simulink model "heading_angle_hold_autopilot"  (R2018b)
settings: Solver=VariableStepAuto  StartTime=0.0  StopTime=40  RelTol=1e-3
values from neighbouring files (symbols this model uses):
  g = 32.2    [heading_angle_hold_autopilot.m]
  V = 876    [heading_angle_hold_autopilot.m]
libraries: cstblocks x1
settings Model: Creator=FARYAL  LastModifiedBy=FARYAL

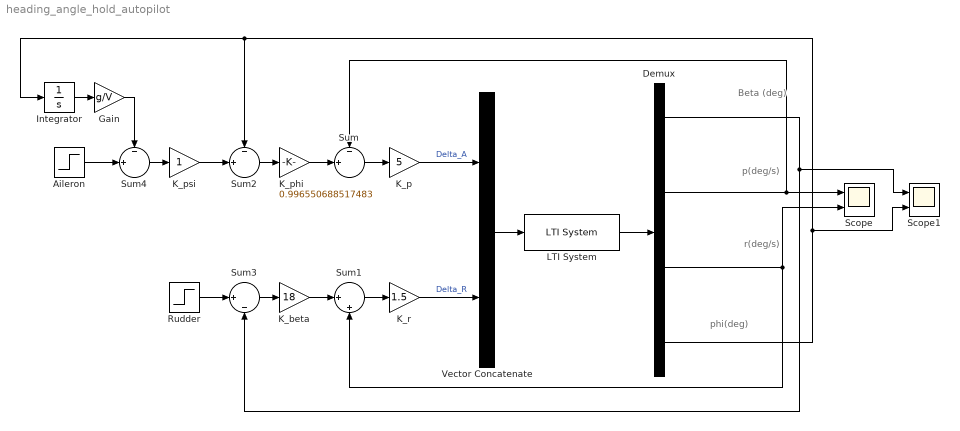
== system heading_angle_hold_autopilot ==
  note: p(deg/s)
  note: phi(deg)
  note: Beta (deg)
  note: r(deg/s)
  "Aileron " : Step  SampleTime=0
  Demux : Demux
  Gain : Gain  Gain=g/V
  Integrator : Integrator
  "K_beta " : Gain  Gain=18
  K_p : Gain  Gain=5
  "K_phi " : Gain  Gain=0.996550688517483
  K_psi : Gain
  "K_r " : Gain  Gain=1.5
  LTI System : cstblocks/LTI System  sys=System  IC=[]
  "Rudder " : Step  After=0  SampleTime=0
  Scope : Scope  NumInputPorts=2
  Scope1 : Scope  NumInputPorts=2
  Sum : Sum  Inputs=-|+||
  Sum1 : Sum  Inputs=||+|+
  Sum2 : Sum  Inputs=-|+||
  Sum3 : Sum  Inputs=||+|-
  Sum4 : Sum  Inputs=-|+||
  Vector Concatenate : Concatenate
  wires:
  "K_r "/1 -> Vector Concatenate/2  "Delta_R"
  LTI System/1 -> Demux/1
  K_p/1 -> Vector Concatenate/1  "Delta_A"
  Demux/3 -> Scope/2, Sum1/2
  "K_phi "/1 -> Sum/2
  Demux/2 -> Sum/1, Scope/1
  Demux/1 -> Sum3/2, Scope1/1
  Sum1/1 -> "K_r "/1
  "K_beta "/1 -> Sum1/1
  Vector Concatenate/1 -> LTI System/1
  "Rudder "/1 -> Sum3/1
  Sum2/1 -> "K_phi "/1
  Demux/4 -> Integrator/1, Sum2/1, Scope1/2
  Sum/1 -> K_p/1
  Sum3/1 -> "K_beta "/1
  K_psi/1 -> Sum2/2
  "Aileron "/1 -> Sum4/2
  Sum4/1 -> K_psi/1
  Gain/1 -> Sum4/1
  Integrator/1 -> Gain/1
